simulink model "hw3"  (R2020a)
settings: Solver=VariableStepAuto  StartTime=0.0  StopTime=1  RelTol=1e-3
undefined symbols (not defined in the file): Beq, D2R, Gr, Jeq, Ka_c, Ka_s, Kd_p, Ke, Ki_c, Ki_s, Kp_c, Kp_p, Kp_s, Kt, La, Ra
(part 1 of 2)
settings Model: Creator=helep  LastModifiedBy=JeongHun Hong
settings SFSimCC: CustomCodeUndefinedFunction=UseInterfaceOnly

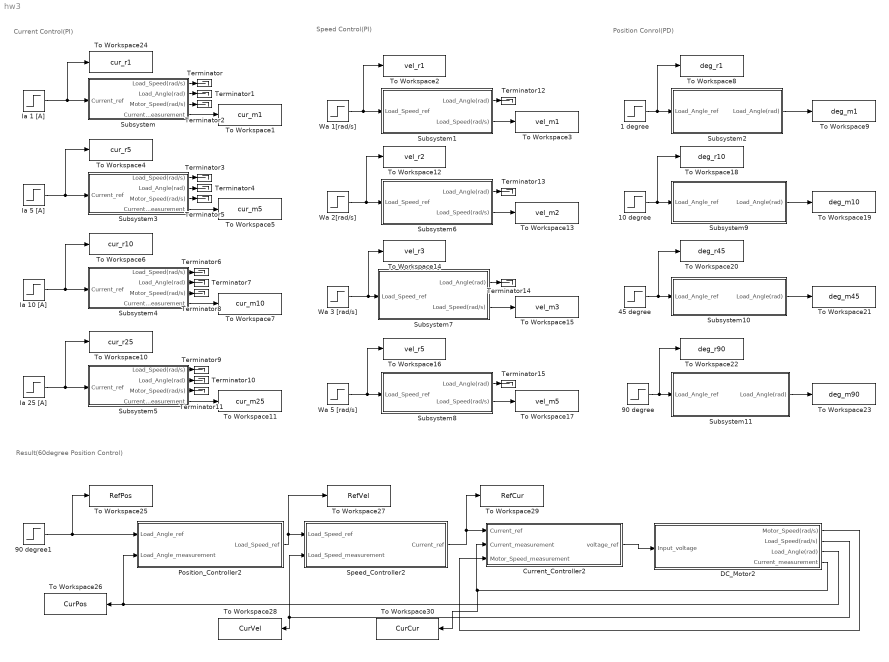
== system hw3 ==
  note: Position Conrol(PD)
  note: Speed Control(PI)
  note: Current Control(PI)
  note: Result(60degree Position Control)
  1 degree : Step  Time=0  After=1*D2R  SampleTime=0
  10 degree : Step  Time=0  After=10*D2R  SampleTime=0
  45 degree : Step  Time=0  After=45*D2R  SampleTime=0
  90 degree : Step  Time=0  After=90*D2R  SampleTime=0
  90 degree1 : Step  Time=0  After=60*D2R  SampleTime=0
  Current_Controller2 : Subsystem
  DC_Motor2 : Subsystem
  Ia 1 [A] : Step  Time=0  SampleTime=0
  Ia 10 [A] : Step  Time=0  After=10  SampleTime=0
  Ia 25 [A] : Step  Time=0  After=25  SampleTime=0
  Ia 5 [A] : Step  Time=0  After=5  SampleTime=0
  Position_Controller2 : Subsystem
  Speed_Controller2 : Subsystem
  Subsystem : Subsystem
  Subsystem1 : Subsystem
  Subsystem10 : Subsystem
  Subsystem11 : Subsystem
  Subsystem2 : Subsystem
  Subsystem3 : Subsystem
  Subsystem4 : Subsystem
  Subsystem5 : Subsystem
  Subsystem6 : Subsystem
  Subsystem7 : Subsystem
  Subsystem8 : Subsystem
  Subsystem9 : Subsystem
  Terminator{,1..15} (16 alike) : Terminator
  To Workspace1 : ToWorkspace  VariableName=cur_m1  SaveFormat=Structure With Time  SampleTime=-1
  To Workspace10 : ToWorkspace  VariableName=cur_r25  SaveFormat=Structure With Time  SampleTime=-1
  To Workspace11 : ToWorkspace  VariableName=cur_m25  SaveFormat=Structure With Time  SampleTime=-1
  To Workspace12 : ToWorkspace  VariableName=vel_r2  SaveFormat=Structure With Time  SampleTime=-1
  To Workspace13 : ToWorkspace  VariableName=vel_m2  SaveFormat=Structure With Time  SampleTime=-1
  To Workspace14 : ToWorkspace  VariableName=vel_r3  SaveFormat=Structure With Time  SampleTime=-1
  To Workspace15 : ToWorkspace  VariableName=vel_m3  SaveFormat=Structure With Time  SampleTime=-1
  To Workspace16 : ToWorkspace  VariableName=vel_r5  SaveFormat=Structure With Time  SampleTime=-1
  To Workspace17 : ToWorkspace  VariableName=vel_m5  SaveFormat=Structure With Time  SampleTime=-1
  To Workspace18 : ToWorkspace  VariableName=deg_r10  SaveFormat=Structure With Time  SampleTime=-1
  To Workspace19 : ToWorkspace  VariableName=deg_m10  SaveFormat=Structure With Time  SampleTime=-1
  To Workspace2 : ToWorkspace  VariableName=vel_r1  SaveFormat=Structure With Time  SampleTime=-1
  To Workspace20 : ToWorkspace  VariableName=deg_r45  SaveFormat=Structure With Time  SampleTime=-1
  To Workspace21 : ToWorkspace  VariableName=deg_m45  SaveFormat=Structure With Time  SampleTime=-1
  To Workspace22 : ToWorkspace  VariableName=deg_r90  SaveFormat=Structure With Time  SampleTime=-1
  To Workspace23 : ToWorkspace  VariableName=deg_m90  SaveFormat=Structure With Time  SampleTime=-1
  To Workspace24 : ToWorkspace  VariableName=cur_r1  SaveFormat=Structure With Time  SampleTime=-1
  To Workspace25 : ToWorkspace  VariableName=RefPos  SaveFormat=Structure With Time  SampleTime=-1
  To Workspace26 : ToWorkspace  VariableName=CurPos  SaveFormat=Structure With Time  SampleTime=-1
  To Workspace27 : ToWorkspace  VariableName=RefVel  SaveFormat=Structure With Time  SampleTime=-1
  To Workspace28 : ToWorkspace  VariableName=CurVel  SaveFormat=Structure With Time  SampleTime=-1
  To Workspace29 : ToWorkspace  VariableName=RefCur  SaveFormat=Structure With Time  SampleTime=-1
  To Workspace3 : ToWorkspace  VariableName=vel_m1  SaveFormat=Structure With Time  SampleTime=-1
  To Workspace30 : ToWorkspace  VariableName=CurCur  SaveFormat=Structure With Time  SampleTime=-1
  To Workspace4 : ToWorkspace  VariableName=cur_r5  SaveFormat=Structure With Time  SampleTime=-1
  To Workspace5 : ToWorkspace  VariableName=cur_m5  SaveFormat=Structure With Time  SampleTime=-1
  To Workspace6 : ToWorkspace  VariableName=cur_r10  SaveFormat=Structure With Time  SampleTime=-1
  To Workspace7 : ToWorkspace  VariableName=cur_m10  SaveFormat=Structure With Time  SampleTime=-1
  To Workspace8 : ToWorkspace  VariableName=deg_r1  SaveFormat=Structure With Time  SampleTime=-1
  To Workspace9 : ToWorkspace  VariableName=deg_m1  SaveFormat=Structure With Time  SampleTime=-1
  Wa 1[rad/s] : Step  Time=0  SampleTime=0
  Wa 2[rad/s] : Step  Time=0  After=2  SampleTime=0
  Wa 3 [rad/s] : Step  Time=0  After=3  SampleTime=0
  Wa 5 [rad/s] : Step  Time=0  After=5  SampleTime=0
  wires:
  Ia 1 [A]/1 -> To Workspace24/1, Subsystem/1(Current_ref)
  Wa 1[rad/s]/1 -> To Workspace2/1, Subsystem1/1(Load_Speed_ref)
  1 degree/1 -> To Workspace8/1, Subsystem2/1(Load_Angle_ref)
  Subsystem1/2(Load_Speed(rad/s)) -> To Workspace3/1
  Subsystem2/1(Load_Angle(rad)) -> To Workspace9/1
  Ia 5 [A]/1 -> To Workspace4/1, Subsystem3/1(Current_ref)
  Ia 10 [A]/1 -> To Workspace6/1, Subsystem4/1(Current_ref)
  Ia 25 [A]/1 -> To Workspace10/1, Subsystem5/1(Current_ref)
  Subsystem6/2(Load_Speed(rad/s)) -> To Workspace13/1
  Wa 2[rad/s]/1 -> To Workspace12/1, Subsystem6/1(Load_Speed_ref)
  Wa 3 [rad/s]/1 -> To Workspace14/1, Subsystem7/1(Load_Speed_ref)
  Wa 5 [rad/s]/1 -> To Workspace16/1, Subsystem8/1(Load_Speed_ref)
  Subsystem7/2(Load_Speed(rad/s)) -> To Workspace15/1
  Subsystem8/2(Load_Speed(rad/s)) -> To Workspace17/1
  10 degree/1 -> To Workspace18/1, Subsystem9/1(Load_Angle_ref)
  45 degree/1 -> To Workspace20/1, Subsystem10/1(Load_Angle_ref)
  90 degree/1 -> To Workspace22/1, Subsystem11/1(Load_Angle_ref)
  Subsystem9/1(Load_Angle(rad)) -> To Workspace19/1
  Subsystem10/1(Load_Angle(rad)) -> To Workspace21/1
  Subsystem11/1(Load_Angle(rad)) -> To Workspace23/1
  Subsystem/4(Current_measurement) -> To Workspace1/1
  Subsystem3/4(Current_measurement) -> To Workspace5/1
  Subsystem4/4(Current_measurement) -> To Workspace7/1
  Subsystem5/4(Current_measurement) -> To Workspace11/1
  Subsystem/1(Load_Speed(rad/s)) -> Terminator/1
  Subsystem/2(Load_Angle(rad)) -> Terminator1/1
  Subsystem/3(Motor_Speed(rad/s)) -> Terminator2/1
  Subsystem1/1(Load_Angle(rad)) -> Terminator12/1
  Subsystem6/1(Load_Angle(rad)) -> Terminator13/1
  Subsystem7/1(Load_Angle(rad)) -> Terminator14/1
  Subsystem8/1(Load_Angle(rad)) -> Terminator15/1
  Subsystem3/1(Load_Speed(rad/s)) -> Terminator3/1
  Subsystem3/2(Load_Angle(rad)) -> Terminator4/1
  Subsystem3/3(Motor_Speed(rad/s)) -> Terminator5/1
  Subsystem4/3(Motor_Speed(rad/s)) -> Terminator8/1
  Subsystem4/2(Load_Angle(rad)) -> Terminator7/1
  Subsystem4/1(Load_Speed(rad/s)) -> Terminator6/1
  Subsystem5/3(Motor_Speed(rad/s)) -> Terminator11/1
  Subsystem5/2(Load_Angle(rad)) -> Terminator10/1
  Subsystem5/1(Load_Speed(rad/s)) -> Terminator9/1
  DC_Motor2/3(Load_Angle(rad)) -> Position_Controller2/2(Load_Angle_measurement), To Workspace26/1
  Current_Controller2/1(voltage_ref) -> DC_Motor2/1(Input_voltage)
  Speed_Controller2/1(Current_ref) -> To Workspace29/1, Current_Controller2/1(Current_ref)
  DC_Motor2/2(Load_Speed(rad/s)) -> To Workspace28/1, Speed_Controller2/2(Load_Speed_measurement)
  DC_Motor2/1(Motor_Speed(rad/s)) -> Current_Controller2/3(Motor_Speed_measurement)
  DC_Motor2/4(Current_measurement) -> To Workspace30/1, Current_Controller2/2(Current_measurement)
  90 degree1/1 -> To Workspace25/1, Position_Controller2/1(Load_Angle_ref)
  Position_Controller2/1(Load_Speed_ref) -> To Workspace27/1, Speed_Controller2/1(Load_Speed_ref)

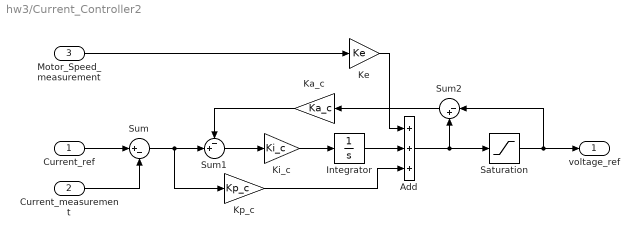
== system hw3/Current_Controller2 ==
  Current_ref : Inport
  Current_measurement : Inport  Port=2
  Motor_Speed_measurement : Inport  Port=3
  Add : Sum  Inputs=+++
  Integrator : Integrator
  Ka_c : Gain  Gain=Ka_c
  Ke : Gain  Gain=Ke
  Ki_c : Gain  Gain=Ki_c
  Kp_c : Gain  Gain=Kp_c
  Saturation : Saturate  UpperLimit=48  LowerLimit=-48
  Sum : Sum  Inputs=|+-
  Sum1 : Sum  Inputs=-+|
  Sum2 : Sum  Inputs=|-+
  voltage_ref : Outport  VectorParamsAs1DForOutWhenUnconnected=off
  wires:
  Saturation/1 -> Sum2/1, voltage_ref/1
  Ke/1 -> Add/1
  Motor_Speed_measurement/1 -> Ke/1
  Ka_c/1 -> Sum1/1
  Current_ref/1 -> Sum/1
  Current_measurement/1 -> Sum/2
  Sum1/1 -> Ki_c/1
  Integrator/1 -> Add/2
  Sum/1 -> Sum1/2, Kp_c/1
  Kp_c/1 -> Add/3
  Sum2/1 -> Ka_c/1
  Ki_c/1 -> Integrator/1
  Add/1 -> Sum2/2, Saturation/1

== system hw3/DC_Motor2 ==
  Input_voltage : Inport
  Back EMF constant1 : Gain  Gain=Ke
  Gr : Gain  Gain=Gr
  Integrator1 : Integrator
  Sum1 : Sum  Inputs=|+-
  Torque constant1 : Gain  Gain=Kt
  Transfer Fcn1 : TransferFcn  Denominator=[La Ra]
  Transfer Fcn3 : TransferFcn  Denominator=[Jeq Beq]
  Motor_Speed(rad/s) : Outport  VectorParamsAs1DForOutWhenUnconnected=off
  Load_Speed(rad/s) : Outport  Port=2  VectorParamsAs1DForOutWhenUnconnected=off
  Load_Angle(rad) : Outport  Port=3  VectorParamsAs1DForOutWhenUnconnected=off
  Current_measurement : Outport  Port=4  VectorParamsAs1DForOutWhenUnconnected=off
  wires:
  Transfer Fcn3/1 -> Back EMF constant1/1, Gr/1, Motor_Speed(rad/s)/1
  Integrator1/1 -> Load_Angle(rad)/1
  Gr/1 -> Integrator1/1, Load_Speed(rad/s)/1
  Input_voltage/1 -> Sum1/1
  Sum1/1 -> Transfer Fcn1/1
  Transfer Fcn1/1 -> Current_measurement/1, Torque constant1/1
  Back EMF constant1/1 -> Sum1/2
  Torque constant1/1 -> Transfer Fcn3/1

== system hw3/Position_Controller2 ==
  Load_Angle_ref : Inport
  Load_Angle_measurement : Inport  Port=2
  Add : Sum
  Derivative : Derivative
  Kd_p : Gain  Gain=Kd_p
  Kp_p : Gain  Gain=Kp_p
  Saturation : Saturate  UpperLimit=6140*pi/30  LowerLimit=-6140*pi/30
  Sum : Sum  Inputs=|+-
  Load_Speed_ref : Outport  VectorParamsAs1DForOutWhenUnconnected=off
  wires:
  Add/1 -> Saturation/1
  Derivative/1 -> Add/2
  Sum/1 -> Kd_p/1, Kp_p/1
  Saturation/1 -> Load_Speed_ref/1
  Kp_p/1 -> Add/1
  Kd_p/1 -> Derivative/1
  Load_Angle_ref/1 -> Sum/1
  Load_Angle_measurement/1 -> Sum/2

== system hw3/Speed_Controller2 ==
  Load_Speed_ref : Inport
  Load_Speed_measurement : Inport  Port=2
  Add : Sum
  Integrator : Integrator
  Ka_s : Gain  Gain=Ka_s
  Ki_s : Gain  Gain=Ki_s
  Kp_s : Gain  Gain=Kp_s
  Saturation : Saturate  UpperLimit=27.3  LowerLimit=-27.3
  Sum : Sum  Inputs=|+-
  Sum1 : Sum  Inputs=-+|
  Sum2 : Sum  Inputs=|-+
  Current_ref : Outport  VectorParamsAs1DForOutWhenUnconnected=off
  wires:
  Integrator/1 -> Add/1
  Sum1/1 -> Ki_s/1
  Ki_s/1 -> Integrator/1
  Saturation/1 -> Sum2/1, Current_ref/1
  Load_Speed_measurement/1 -> Sum/2
  Ka_s/1 -> Sum1/1
  Sum2/1 -> Ka_s/1
  Add/1 -> Saturation/1, Sum2/2
  Load_Speed_ref/1 -> Sum/1
  Kp_s/1 -> Add/2
  Sum/1 -> Sum1/2, Kp_s/1

== system hw3/Subsystem ==
  Current_ref : Inport
  Current_Controller : Subsystem
  DC_Motor : Subsystem
  Load_Speed(rad/s) : Outport
  Load_Angle(rad) : Outport  Port=2
  Motor_Speed(rad/s) : Outport  Port=3
  Current_measurement : Outport  Port=4
  wires:
  DC_Motor/1(Motor_Speed(rad/s)) -> Motor_Speed(rad/s)/1, Current_Controller/3(Motor_Speed_measurement)
  Current_ref/1 -> Current_Controller/1(Current_ref)
  DC_Motor/2(Load_Speed(rad/s)) -> Load_Speed(rad/s)/1
  Current_Controller/1(voltage_ref) -> DC_Motor/1(Input_voltage)
  DC_Motor/3(Load_Angle(rad)) -> Load_Angle(rad)/1
  DC_Motor/4(Current_measurement) -> Current_measurement/1, Current_Controller/2(Current_measurement)

== system hw3/Subsystem1 ==
  Load_Speed_ref : Inport
  Current_Controller1 : Subsystem
  DC_Motor1 : Subsystem
  Speed_Controller1 : Subsystem
  Load_Angle(rad) : Outport
  Load_Speed(rad/s) : Outport  Port=2
  wires:
  Current_Controller1/1(voltage_ref) -> DC_Motor1/1(Input_voltage)
  DC_Motor1/2(Load_Speed(rad/s)) -> Load_Speed(rad/s)/1, Speed_Controller1/2(Load_Speed_measurement)
  Speed_Controller1/1(Current_ref) -> Current_Controller1/1(Current_ref)
  Load_Speed_ref/1 -> Speed_Controller1/1(Load_Speed_ref)
  DC_Motor1/3(Load_Angle(rad)) -> Load_Angle(rad)/1
  DC_Motor1/4(Current_measurement) -> Current_Controller1/2(Current_measurement)
  DC_Motor1/1(Motor_Speed(rad/s)) -> Current_Controller1/3(Motor_Speed_measurement)

== system hw3/Subsystem10 ==
  Load_Angle_ref : Inport
  Current_Controller2 : Subsystem
  DC_Motor2 : Subsystem
  Position_Controller2 : Subsystem
  Speed_Controller2 : Subsystem
  Load_Angle(rad) : Outport
  wires:
  DC_Motor2/3(Load_Angle(rad)) -> Load_Angle(rad)/1, Position_Controller2/2(Load_Angle_measurement)
  Load_Angle_ref/1 -> Position_Controller2/1(Load_Angle_ref)
  Current_Controller2/1(voltage_ref) -> DC_Motor2/1(Input_voltage)
  Speed_Controller2/1(Current_ref) -> Current_Controller2/1(Current_ref)
  DC_Motor2/2(Load_Speed(rad/s)) -> Speed_Controller2/2(Load_Speed_measurement)
  Position_Controller2/1(Load_Speed_ref) -> Speed_Controller2/1(Load_Speed_ref)
  DC_Motor2/1(Motor_Speed(rad/s)) -> Current_Controller2/3(Motor_Speed_measurement)
  DC_Motor2/4(Current_measurement) -> Current_Controller2/2(Current_measurement)

== system hw3/Subsystem11 ==
  Load_Angle_ref : Inport
  Current_Controller2 : Subsystem
  DC_Motor2 : Subsystem
  Position_Controller2 : Subsystem
  Speed_Controller2 : Subsystem
  Load_Angle(rad) : Outport
  wires:
  DC_Motor2/4(Current_measurement) -> Current_Controller2/2(Current_measurement)
  DC_Motor2/1(Motor_Speed(rad/s)) -> Current_Controller2/3(Motor_Speed_measurement)
  Position_Controller2/1(Load_Speed_ref) -> Speed_Controller2/1(Load_Speed_ref)
  DC_Motor2/2(Load_Speed(rad/s)) -> Speed_Controller2/2(Load_Speed_measurement)
  Speed_Controller2/1(Current_ref) -> Current_Controller2/1(Current_ref)
  Current_Controller2/1(voltage_ref) -> DC_Motor2/1(Input_voltage)
  Load_Angle_ref/1 -> Position_Controller2/1(Load_Angle_ref)
  DC_Motor2/3(Load_Angle(rad)) -> Position_Controller2/2(Load_Angle_measurement), Load_Angle(rad)/1

== system hw3/Subsystem2 ==
  Load_Angle_ref : Inport
  Current_Controller2 : Subsystem
  DC_Motor2 : Subsystem
  Position_Controller2 : Subsystem
  Speed_Controller2 : Subsystem
  Load_Angle(rad) : Outport
  wires:
  DC_Motor2/3(Load_Angle(rad)) -> Load_Angle(rad)/1, Position_Controller2/2(Load_Angle_measurement)
  Load_Angle_ref/1 -> Position_Controller2/1(Load_Angle_ref)
  Current_Controller2/1(voltage_ref) -> DC_Motor2/1(Input_voltage)
  Speed_Controller2/1(Current_ref) -> Current_Controller2/1(Current_ref)
  DC_Motor2/2(Load_Speed(rad/s)) -> Speed_Controller2/2(Load_Speed_measurement)
  Position_Controller2/1(Load_Speed_ref) -> Speed_Controller2/1(Load_Speed_ref)
  DC_Motor2/1(Motor_Speed(rad/s)) -> Current_Controller2/3(Motor_Speed_measurement)
  DC_Motor2/4(Current_measurement) -> Current_Controller2/2(Current_measurement)

== system hw3/Subsystem3 ==
  Current_ref : Inport
  Current_Controller : Subsystem
  DC_Motor : Subsystem
  Load_Speed(rad/s) : Outport
  Load_Angle(rad) : Outport  Port=2
  Motor_Speed(rad/s) : Outport  Port=3
  Current_measurement : Outport  Port=4
  wires:
  DC_Motor/4(Current_measurement) -> Current_measurement/1, Current_Controller/2(Current_measurement)
  DC_Motor/3(Load_Angle(rad)) -> Load_Angle(rad)/1
  Current_Controller/1(voltage_ref) -> DC_Motor/1(Input_voltage)
  DC_Motor/2(Load_Speed(rad/s)) -> Load_Speed(rad/s)/1
  Current_ref/1 -> Current_Controller/1(Current_ref)
  DC_Motor/1(Motor_Speed(rad/s)) -> Current_Controller/3(Motor_Speed_measurement), Motor_Speed(rad/s)/1

== system hw3/Subsystem4 ==
  Current_ref : Inport
  Current_Controller : Subsystem
  DC_Motor : Subsystem
  Load_Speed(rad/s) : Outport
  Load_Angle(rad) : Outport  Port=2
  Motor_Speed(rad/s) : Outport  Port=3
  Current_measurement : Outport  Port=4
  wires:
  DC_Motor/1(Motor_Speed(rad/s)) -> Motor_Speed(rad/s)/1, Current_Controller/3(Motor_Speed_measurement)
  Current_ref/1 -> Current_Controller/1(Current_ref)
  DC_Motor/2(Load_Speed(rad/s)) -> Load_Speed(rad/s)/1
  Current_Controller/1(voltage_ref) -> DC_Motor/1(Input_voltage)
  DC_Motor/3(Load_Angle(rad)) -> Load_Angle(rad)/1
  DC_Motor/4(Current_measurement) -> Current_measurement/1, Current_Controller/2(Current_measurement)

== system hw3/Subsystem5 ==
  Current_ref : Inport
  Current_Controller : Subsystem
  DC_Motor : Subsystem
  Load_Speed(rad/s) : Outport
  Load_Angle(rad) : Outport  Port=2
  Motor_Speed(rad/s) : Outport  Port=3
  Current_measurement : Outport  Port=4
  wires:
  DC_Motor/4(Current_measurement) -> Current_measurement/1, Current_Controller/2(Current_measurement)
  DC_Motor/3(Load_Angle(rad)) -> Load_Angle(rad)/1
  Current_Controller/1(voltage_ref) -> DC_Motor/1(Input_voltage)
  DC_Motor/2(Load_Speed(rad/s)) -> Load_Speed(rad/s)/1
  Current_ref/1 -> Current_Controller/1(Current_ref)
  DC_Motor/1(Motor_Speed(rad/s)) -> Current_Controller/3(Motor_Speed_measurement), Motor_Speed(rad/s)/1

== system hw3/Subsystem6 ==
  Load_Speed_ref : Inport
  Current_Controller1 : Subsystem
  DC_Motor1 : Subsystem
  Speed_Controller1 : Subsystem
  Load_Angle(rad) : Outport
  Load_Speed(rad/s) : Outport  Port=2
  wires:
  DC_Motor1/1(Motor_Speed(rad/s)) -> Current_Controller1/3(Motor_Speed_measurement)
  DC_Motor1/4(Current_measurement) -> Current_Controller1/2(Current_measurement)
  DC_Motor1/3(Load_Angle(rad)) -> Load_Angle(rad)/1
  Load_Speed_ref/1 -> Speed_Controller1/1(Load_Speed_ref)
  Speed_Controller1/1(Current_ref) -> Current_Controller1/1(Current_ref)
  DC_Motor1/2(Load_Speed(rad/s)) -> Speed_Controller1/2(Load_Speed_measurement), Load_Speed(rad/s)/1
  Current_Controller1/1(voltage_ref) -> DC_Motor1/1(Input_voltage)

== system hw3/Subsystem7 ==
  Load_Speed_ref : Inport
  Current_Controller1 : Subsystem
  DC_Motor1 : Subsystem
  Speed_Controller1 : Subsystem
  Load_Angle(rad) : Outport
  Load_Speed(rad/s) : Outport  Port=2
  wires:
  Current_Controller1/1(voltage_ref) -> DC_Motor1/1(Input_voltage)
  DC_Motor1/2(Load_Speed(rad/s)) -> Load_Speed(rad/s)/1, Speed_Controller1/2(Load_Speed_measurement)
  Speed_Controller1/1(Current_ref) -> Current_Controller1/1(Current_ref)
  Load_Speed_ref/1 -> Speed_Controller1/1(Load_Speed_ref)
  DC_Motor1/3(Load_Angle(rad)) -> Load_Angle(rad)/1
  DC_Motor1/4(Current_measurement) -> Current_Controller1/2(Current_measurement)
  DC_Motor1/1(Motor_Speed(rad/s)) -> Current_Controller1/3(Motor_Speed_measurement)

== system hw3/Subsystem8 ==
  Load_Speed_ref : Inport
  Current_Controller1 : Subsystem
  DC_Motor1 : Subsystem
  Speed_Controller1 : Subsystem
  Load_Angle(rad) : Outport
  Load_Speed(rad/s) : Outport  Port=2
  wires:
  DC_Motor1/1(Motor_Speed(rad/s)) -> Current_Controller1/3(Motor_Speed_measurement)
  DC_Motor1/4(Current_measurement) -> Current_Controller1/2(Current_measurement)
  DC_Motor1/3(Load_Angle(rad)) -> Load_Angle(rad)/1
  Load_Speed_ref/1 -> Speed_Controller1/1(Load_Speed_ref)
  Speed_Controller1/1(Current_ref) -> Current_Controller1/1(Current_ref)
  DC_Motor1/2(Load_Speed(rad/s)) -> Speed_Controller1/2(Load_Speed_measurement), Load_Speed(rad/s)/1
  Current_Controller1/1(voltage_ref) -> DC_Motor1/1(Input_voltage)

== system hw3/Subsystem9 ==
  Load_Angle_ref : Inport
  Current_Controller2 : Subsystem
  DC_Motor2 : Subsystem
  Position_Controller2 : Subsystem
  Speed_Controller2 : Subsystem
  Load_Angle(rad) : Outport
  wires:
  DC_Motor2/4(Current_measurement) -> Current_Controller2/2(Current_measurement)
  DC_Motor2/1(Motor_Speed(rad/s)) -> Current_Controller2/3(Motor_Speed_measurement)
  Position_Controller2/1(Load_Speed_ref) -> Speed_Controller2/1(Load_Speed_ref)
  DC_Motor2/2(Load_Speed(rad/s)) -> Speed_Controller2/2(Load_Speed_measurement)
  Speed_Controller2/1(Current_ref) -> Current_Controller2/1(Current_ref)
  Current_Controller2/1(voltage_ref) -> DC_Motor2/1(Input_voltage)
  Load_Angle_ref/1 -> Position_Controller2/1(Load_Angle_ref)
  DC_Motor2/3(Load_Angle(rad)) -> Position_Controller2/2(Load_Angle_measurement), Load_Angle(rad)/1

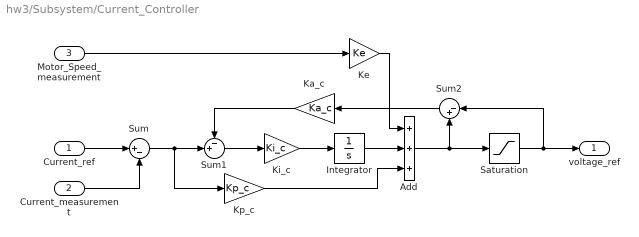
== system hw3/Subsystem/Current_Controller ==
  Current_ref : Inport
  Current_measurement : Inport  Port=2
  Motor_Speed_measurement : Inport  Port=3
  Add : Sum  Inputs=+++
  Integrator : Integrator
  Ka_c : Gain  Gain=Ka_c
  Ke : Gain  Gain=Ke
  Ki_c : Gain  Gain=Ki_c
  Kp_c : Gain  Gain=Kp_c
  Saturation : Saturate  UpperLimit=48  LowerLimit=-48
  Sum : Sum  Inputs=|+-
  Sum1 : Sum  Inputs=-+|
  Sum2 : Sum  Inputs=|-+
  voltage_ref : Outport  VectorParamsAs1DForOutWhenUnconnected=off
  wires:
  Add/1 -> Saturation/1, Sum2/2
  Ki_c/1 -> Integrator/1
  Sum2/1 -> Ka_c/1
  Kp_c/1 -> Add/3
  Sum/1 -> Kp_c/1, Sum1/2
  Integrator/1 -> Add/2
  Sum1/1 -> Ki_c/1
  Current_measurement/1 -> Sum/2
  Current_ref/1 -> Sum/1
  Ka_c/1 -> Sum1/1
  Motor_Speed_measurement/1 -> Ke/1
  Ke/1 -> Add/1
  Saturation/1 -> voltage_ref/1, Sum2/1

== system hw3/Subsystem/DC_Motor ==
  Input_voltage : Inport
  Back EMF constant1 : Gain  Gain=Ke
  Gr : Gain  Gain=Gr
  Integrator1 : Integrator
  Sum1 : Sum  Inputs=|+-
  Torque constant1 : Gain  Gain=Kt
  Transfer Fcn1 : TransferFcn  Denominator=[La Ra]
  Transfer Fcn3 : TransferFcn  Denominator=[Jeq Beq]
  Motor_Speed(rad/s) : Outport  VectorParamsAs1DForOutWhenUnconnected=off
  Load_Speed(rad/s) : Outport  Port=2  VectorParamsAs1DForOutWhenUnconnected=off
  Load_Angle(rad) : Outport  Port=3  VectorParamsAs1DForOutWhenUnconnected=off
  Current_measurement : Outport  Port=4  VectorParamsAs1DForOutWhenUnconnected=off
  wires:
  Torque constant1/1 -> Transfer Fcn3/1
  Back EMF constant1/1 -> Sum1/2
  Transfer Fcn1/1 -> Torque constant1/1, Current_measurement/1
  Sum1/1 -> Transfer Fcn1/1
  Input_voltage/1 -> Sum1/1
  Gr/1 -> Load_Speed(rad/s)/1, Integrator1/1
  Integrator1/1 -> Load_Angle(rad)/1
  Transfer Fcn3/1 -> Motor_Speed(rad/s)/1, Gr/1, Back EMF constant1/1

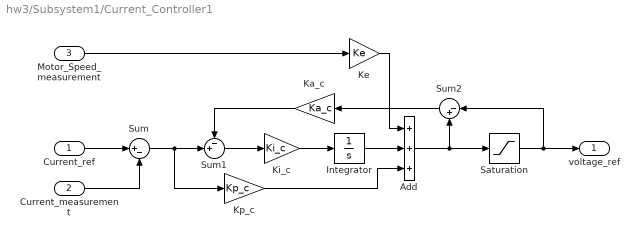
== system hw3/Subsystem1/Current_Controller1 ==
  Current_ref : Inport
  Current_measurement : Inport  Port=2
  Motor_Speed_measurement : Inport  Port=3
  Add : Sum  Inputs=+++
  Integrator : Integrator
  Ka_c : Gain  Gain=Ka_c
  Ke : Gain  Gain=Ke
  Ki_c : Gain  Gain=Ki_c
  Kp_c : Gain  Gain=Kp_c
  Saturation : Saturate  UpperLimit=48  LowerLimit=-48
  Sum : Sum  Inputs=|+-
  Sum1 : Sum  Inputs=-+|
  Sum2 : Sum  Inputs=|-+
  voltage_ref : Outport  VectorParamsAs1DForOutWhenUnconnected=off
  wires:
  Saturation/1 -> Sum2/1, voltage_ref/1
  Ke/1 -> Add/1
  Motor_Speed_measurement/1 -> Ke/1
  Ka_c/1 -> Sum1/1
  Current_ref/1 -> Sum/1
  Current_measurement/1 -> Sum/2
  Sum1/1 -> Ki_c/1
  Integrator/1 -> Add/2
  Sum/1 -> Sum1/2, Kp_c/1
  Kp_c/1 -> Add/3
  Sum2/1 -> Ka_c/1
  Ki_c/1 -> Integrator/1
  Add/1 -> Sum2/2, Saturation/1

== system hw3/Subsystem1/DC_Motor1 ==
  Input_voltage : Inport
  Back EMF constant1 : Gain  Gain=Ke
  Gr : Gain  Gain=Gr
  Integrator1 : Integrator
  Sum1 : Sum  Inputs=|+-
  Torque constant1 : Gain  Gain=Kt
  Transfer Fcn1 : TransferFcn  Denominator=[La Ra]
  Transfer Fcn3 : TransferFcn  Denominator=[Jeq Beq]
  Motor_Speed(rad/s) : Outport  VectorParamsAs1DForOutWhenUnconnected=off
  Load_Speed(rad/s) : Outport  Port=2  VectorParamsAs1DForOutWhenUnconnected=off
  Load_Angle(rad) : Outport  Port=3  VectorParamsAs1DForOutWhenUnconnected=off
  Current_measurement : Outport  Port=4  VectorParamsAs1DForOutWhenUnconnected=off
  wires:
  Transfer Fcn3/1 -> Back EMF constant1/1, Gr/1, Motor_Speed(rad/s)/1
  Integrator1/1 -> Load_Angle(rad)/1
  Gr/1 -> Integrator1/1, Load_Speed(rad/s)/1
  Input_voltage/1 -> Sum1/1
  Sum1/1 -> Transfer Fcn1/1
  Transfer Fcn1/1 -> Current_measurement/1, Torque constant1/1
  Back EMF constant1/1 -> Sum1/2
  Torque constant1/1 -> Transfer Fcn3/1

== system hw3/Subsystem1/Speed_Controller1 ==
  Load_Speed_ref : Inport
  Load_Speed_measurement : Inport  Port=2
  Add : Sum
  Integrator : Integrator
  Ka_s : Gain  Gain=Ka_s
  Ki_s : Gain  Gain=Ki_s
  Kp_s : Gain  Gain=Kp_s
  Saturation : Saturate  UpperLimit=27.3  LowerLimit=-27.3
  Sum : Sum  Inputs=|+-
  Sum1 : Sum  Inputs=-+|
  Sum2 : Sum  Inputs=|-+
  Current_ref : Outport  VectorParamsAs1DForOutWhenUnconnected=off
  wires:
  Integrator/1 -> Add/1
  Sum1/1 -> Ki_s/1
  Ki_s/1 -> Integrator/1
  Saturation/1 -> Sum2/1, Current_ref/1
  Load_Speed_measurement/1 -> Sum/2
  Ka_s/1 -> Sum1/1
  Sum2/1 -> Ka_s/1
  Add/1 -> Saturation/1, Sum2/2
  Load_Speed_ref/1 -> Sum/1
  Kp_s/1 -> Add/2
  Sum/1 -> Sum1/2, Kp_s/1

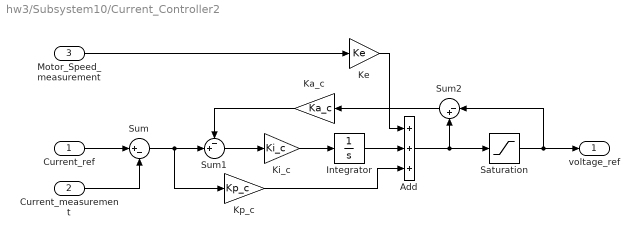
== system hw3/Subsystem10/Current_Controller2 ==
  Current_ref : Inport
  Current_measurement : Inport  Port=2
  Motor_Speed_measurement : Inport  Port=3
  Add : Sum  Inputs=+++
  Integrator : Integrator
  Ka_c : Gain  Gain=Ka_c
  Ke : Gain  Gain=Ke
  Ki_c : Gain  Gain=Ki_c
  Kp_c : Gain  Gain=Kp_c
  Saturation : Saturate  UpperLimit=48  LowerLimit=-48
  Sum : Sum  Inputs=|+-
  Sum1 : Sum  Inputs=-+|
  Sum2 : Sum  Inputs=|-+
  voltage_ref : Outport  VectorParamsAs1DForOutWhenUnconnected=off
  wires:
  Add/1 -> Saturation/1, Sum2/2
  Ki_c/1 -> Integrator/1
  Sum2/1 -> Ka_c/1
  Kp_c/1 -> Add/3
  Sum/1 -> Kp_c/1, Sum1/2
  Integrator/1 -> Add/2
  Sum1/1 -> Ki_c/1
  Current_measurement/1 -> Sum/2
  Current_ref/1 -> Sum/1
  Ka_c/1 -> Sum1/1
  Motor_Speed_measurement/1 -> Ke/1
  Ke/1 -> Add/1
  Saturation/1 -> voltage_ref/1, Sum2/1

== system hw3/Subsystem10/DC_Motor2 ==
  Input_voltage : Inport
  Back EMF constant1 : Gain  Gain=Ke
  Gr : Gain  Gain=Gr
  Integrator1 : Integrator
  Sum1 : Sum  Inputs=|+-
  Torque constant1 : Gain  Gain=Kt
  Transfer Fcn1 : TransferFcn  Denominator=[La Ra]
  Transfer Fcn3 : TransferFcn  Denominator=[Jeq Beq]
  Motor_Speed(rad/s) : Outport  VectorParamsAs1DForOutWhenUnconnected=off
  Load_Speed(rad/s) : Outport  Port=2  VectorParamsAs1DForOutWhenUnconnected=off
  Load_Angle(rad) : Outport  Port=3  VectorParamsAs1DForOutWhenUnconnected=off
  Current_measurement : Outport  Port=4  VectorParamsAs1DForOutWhenUnconnected=off
  wires:
  Torque constant1/1 -> Transfer Fcn3/1
  Back EMF constant1/1 -> Sum1/2
  Transfer Fcn1/1 -> Torque constant1/1, Current_measurement/1
  Sum1/1 -> Transfer Fcn1/1
  Input_voltage/1 -> Sum1/1
  Gr/1 -> Load_Speed(rad/s)/1, Integrator1/1
  Integrator1/1 -> Load_Angle(rad)/1
  Transfer Fcn3/1 -> Motor_Speed(rad/s)/1, Gr/1, Back EMF constant1/1

== system hw3/Subsystem10/Position_Controller2 ==
  Load_Angle_ref : Inport
  Load_Angle_measurement : Inport  Port=2
  Add : Sum
  Derivative : Derivative
  Kd_p : Gain  Gain=Kd_p
  Kp_p : Gain  Gain=Kp_p
  Saturation : Saturate  UpperLimit=6140*pi/30  LowerLimit=-6140*pi/30
  Sum : Sum  Inputs=|+-
  Load_Speed_ref : Outport  VectorParamsAs1DForOutWhenUnconnected=off
  wires:
  Load_Angle_measurement/1 -> Sum/2
  Load_Angle_ref/1 -> Sum/1
  Kd_p/1 -> Derivative/1
  Kp_p/1 -> Add/1
  Saturation/1 -> Load_Speed_ref/1
  Sum/1 -> Kp_p/1, Kd_p/1
  Derivative/1 -> Add/2
  Add/1 -> Saturation/1

== system hw3/Subsystem10/Speed_Controller2 ==
  Load_Speed_ref : Inport
  Load_Speed_measurement : Inport  Port=2
  Add : Sum
  Integrator : Integrator
  Ka_s : Gain  Gain=Ka_s
  Ki_s : Gain  Gain=Ki_s
  Kp_s : Gain  Gain=Kp_s
  Saturation : Saturate  UpperLimit=27.3  LowerLimit=-27.3
  Sum : Sum  Inputs=|+-
  Sum1 : Sum  Inputs=-+|
  Sum2 : Sum  Inputs=|-+
  Current_ref : Outport  VectorParamsAs1DForOutWhenUnconnected=off
  wires:
  Sum/1 -> Kp_s/1, Sum1/2
  Kp_s/1 -> Add/2
  Load_Speed_ref/1 -> Sum/1
  Add/1 -> Sum2/2, Saturation/1
  Sum2/1 -> Ka_s/1
  Ka_s/1 -> Sum1/1
  Load_Speed_measurement/1 -> Sum/2
  Saturation/1 -> Current_ref/1, Sum2/1
  Ki_s/1 -> Integrator/1
  Sum1/1 -> Ki_s/1
  Integrator/1 -> Add/1

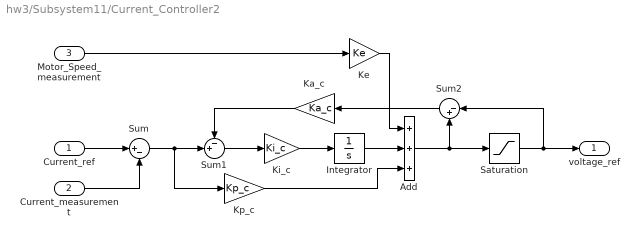
== system hw3/Subsystem11/Current_Controller2 ==
  Current_ref : Inport
  Current_measurement : Inport  Port=2
  Motor_Speed_measurement : Inport  Port=3
  Add : Sum  Inputs=+++
  Integrator : Integrator
  Ka_c : Gain  Gain=Ka_c
  Ke : Gain  Gain=Ke
  Ki_c : Gain  Gain=Ki_c
  Kp_c : Gain  Gain=Kp_c
  Saturation : Saturate  UpperLimit=48  LowerLimit=-48
  Sum : Sum  Inputs=|+-
  Sum1 : Sum  Inputs=-+|
  Sum2 : Sum  Inputs=|-+
  voltage_ref : Outport  VectorParamsAs1DForOutWhenUnconnected=off
  wires:
  Saturation/1 -> Sum2/1, voltage_ref/1
  Ke/1 -> Add/1
  Motor_Speed_measurement/1 -> Ke/1
  Ka_c/1 -> Sum1/1
  Current_ref/1 -> Sum/1
  Current_measurement/1 -> Sum/2
  Sum1/1 -> Ki_c/1
  Integrator/1 -> Add/2
  Sum/1 -> Sum1/2, Kp_c/1
  Kp_c/1 -> Add/3
  Sum2/1 -> Ka_c/1
  Ki_c/1 -> Integrator/1
  Add/1 -> Sum2/2, Saturation/1

== system hw3/Subsystem11/DC_Motor2 ==
  Input_voltage : Inport
  Back EMF constant1 : Gain  Gain=Ke
  Gr : Gain  Gain=Gr
  Integrator1 : Integrator
  Sum1 : Sum  Inputs=|+-
  Torque constant1 : Gain  Gain=Kt
  Transfer Fcn1 : TransferFcn  Denominator=[La Ra]
  Transfer Fcn3 : TransferFcn  Denominator=[Jeq Beq]
  Motor_Speed(rad/s) : Outport  VectorParamsAs1DForOutWhenUnconnected=off
  Load_Speed(rad/s) : Outport  Port=2  VectorParamsAs1DForOutWhenUnconnected=off
  Load_Angle(rad) : Outport  Port=3  VectorParamsAs1DForOutWhenUnconnected=off
  Current_measurement : Outport  Port=4  VectorParamsAs1DForOutWhenUnconnected=off
  wires:
  Transfer Fcn3/1 -> Back EMF constant1/1, Gr/1, Motor_Speed(rad/s)/1
  Integrator1/1 -> Load_Angle(rad)/1
  Gr/1 -> Integrator1/1, Load_Speed(rad/s)/1
  Input_voltage/1 -> Sum1/1
  Sum1/1 -> Transfer Fcn1/1
  Transfer Fcn1/1 -> Current_measurement/1, Torque constant1/1
  Back EMF constant1/1 -> Sum1/2
  Torque constant1/1 -> Transfer Fcn3/1

== system hw3/Subsystem11/Position_Controller2 ==
  Load_Angle_ref : Inport
  Load_Angle_measurement : Inport  Port=2
  Add : Sum
  Derivative : Derivative
  Kd_p : Gain  Gain=Kd_p
  Kp_p : Gain  Gain=Kp_p
  Saturation : Saturate  UpperLimit=6140*pi/30  LowerLimit=-6140*pi/30
  Sum : Sum  Inputs=|+-
  Load_Speed_ref : Outport  VectorParamsAs1DForOutWhenUnconnected=off
  wires:
  Add/1 -> Saturation/1
  Derivative/1 -> Add/2
  Sum/1 -> Kd_p/1, Kp_p/1
  Saturation/1 -> Load_Speed_ref/1
  Kp_p/1 -> Add/1
  Kd_p/1 -> Derivative/1
  Load_Angle_ref/1 -> Sum/1
  Load_Angle_measurement/1 -> Sum/2

== system hw3/Subsystem11/Speed_Controller2 ==
  Load_Speed_ref : Inport
  Load_Speed_measurement : Inport  Port=2
  Add : Sum
  Integrator : Integrator
  Ka_s : Gain  Gain=Ka_s
  Ki_s : Gain  Gain=Ki_s
  Kp_s : Gain  Gain=Kp_s
  Saturation : Saturate  UpperLimit=27.3  LowerLimit=-27.3
  Sum : Sum  Inputs=|+-
  Sum1 : Sum  Inputs=-+|
  Sum2 : Sum  Inputs=|-+
  Current_ref : Outport  VectorParamsAs1DForOutWhenUnconnected=off
  wires:
  Integrator/1 -> Add/1
  Sum1/1 -> Ki_s/1
  Ki_s/1 -> Integrator/1
  Saturation/1 -> Sum2/1, Current_ref/1
  Load_Speed_measurement/1 -> Sum/2
  Ka_s/1 -> Sum1/1
  Sum2/1 -> Ka_s/1
  Add/1 -> Saturation/1, Sum2/2
  Load_Speed_ref/1 -> Sum/1
  Kp_s/1 -> Add/2
  Sum/1 -> Sum1/2, Kp_s/1

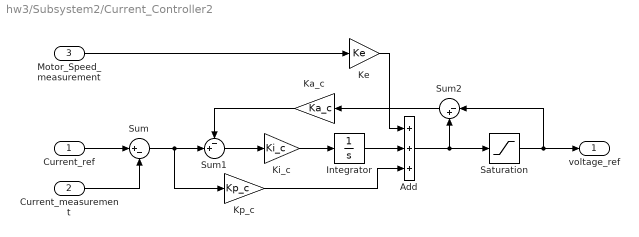
== system hw3/Subsystem2/Current_Controller2 ==
  Current_ref : Inport
  Current_measurement : Inport  Port=2
  Motor_Speed_measurement : Inport  Port=3
  Add : Sum  Inputs=+++
  Integrator : Integrator
  Ka_c : Gain  Gain=Ka_c
  Ke : Gain  Gain=Ke
  Ki_c : Gain  Gain=Ki_c
  Kp_c : Gain  Gain=Kp_c
  Saturation : Saturate  UpperLimit=48  LowerLimit=-48
  Sum : Sum  Inputs=|+-
  Sum1 : Sum  Inputs=-+|
  Sum2 : Sum  Inputs=|-+
  voltage_ref : Outport  VectorParamsAs1DForOutWhenUnconnected=off
  wires:
  Add/1 -> Saturation/1, Sum2/2
  Ki_c/1 -> Integrator/1
  Sum2/1 -> Ka_c/1
  Kp_c/1 -> Add/3
  Sum/1 -> Kp_c/1, Sum1/2
  Integrator/1 -> Add/2
  Sum1/1 -> Ki_c/1
  Current_measurement/1 -> Sum/2
  Current_ref/1 -> Sum/1
  Ka_c/1 -> Sum1/1
  Motor_Speed_measurement/1 -> Ke/1
  Ke/1 -> Add/1
  Saturation/1 -> voltage_ref/1, Sum2/1

== system hw3/Subsystem2/DC_Motor2 ==
  Input_voltage : Inport
  Back EMF constant1 : Gain  Gain=Ke
  Gr : Gain  Gain=Gr
  Integrator1 : Integrator
  Sum1 : Sum  Inputs=|+-
  Torque constant1 : Gain  Gain=Kt
  Transfer Fcn1 : TransferFcn  Denominator=[La Ra]
  Transfer Fcn3 : TransferFcn  Denominator=[Jeq Beq]
  Motor_Speed(rad/s) : Outport  VectorParamsAs1DForOutWhenUnconnected=off
  Load_Speed(rad/s) : Outport  Port=2  VectorParamsAs1DForOutWhenUnconnected=off
  Load_Angle(rad) : Outport  Port=3  VectorParamsAs1DForOutWhenUnconnected=off
  Current_measurement : Outport  Port=4  VectorParamsAs1DForOutWhenUnconnected=off
  wires:
  Torque constant1/1 -> Transfer Fcn3/1
  Back EMF constant1/1 -> Sum1/2
  Transfer Fcn1/1 -> Torque constant1/1, Current_measurement/1
  Sum1/1 -> Transfer Fcn1/1
  Input_voltage/1 -> Sum1/1
  Gr/1 -> Load_Speed(rad/s)/1, Integrator1/1
  Integrator1/1 -> Load_Angle(rad)/1
  Transfer Fcn3/1 -> Motor_Speed(rad/s)/1, Gr/1, Back EMF constant1/1

== system hw3/Subsystem2/Position_Controller2 ==
  Load_Angle_ref : Inport
  Load_Angle_measurement : Inport  Port=2
  Add : Sum
  Derivative : Derivative
  Kd_p : Gain  Gain=Kd_p
  Kp_p : Gain  Gain=Kp_p
  Saturation : Saturate  UpperLimit=6140*pi/30  LowerLimit=-6140*pi/30
  Sum : Sum  Inputs=|+-
  Load_Speed_ref : Outport  VectorParamsAs1DForOutWhenUnconnected=off
  wires:
  Load_Angle_measurement/1 -> Sum/2
  Load_Angle_ref/1 -> Sum/1
  Kd_p/1 -> Derivative/1
  Kp_p/1 -> Add/1
  Saturation/1 -> Load_Speed_ref/1
  Sum/1 -> Kp_p/1, Kd_p/1
  Derivative/1 -> Add/2
  Add/1 -> Saturation/1

== system hw3/Subsystem2/Speed_Controller2 ==
  Load_Speed_ref : Inport
  Load_Speed_measurement : Inport  Port=2
  Add : Sum
  Integrator : Integrator
  Ka_s : Gain  Gain=Ka_s
  Ki_s : Gain  Gain=Ki_s
  Kp_s : Gain  Gain=Kp_s
  Saturation : Saturate  UpperLimit=27.3  LowerLimit=-27.3
  Sum : Sum  Inputs=|+-
  Sum1 : Sum  Inputs=-+|
  Sum2 : Sum  Inputs=|-+
  Current_ref : Outport  VectorParamsAs1DForOutWhenUnconnected=off
  wires:
  Sum/1 -> Kp_s/1, Sum1/2
  Kp_s/1 -> Add/2
  Load_Speed_ref/1 -> Sum/1
  Add/1 -> Sum2/2, Saturation/1
  Sum2/1 -> Ka_s/1
  Ka_s/1 -> Sum1/1
  Load_Speed_measurement/1 -> Sum/2
  Saturation/1 -> Current_ref/1, Sum2/1
  Ki_s/1 -> Integrator/1
  Sum1/1 -> Ki_s/1
  Integrator/1 -> Add/1

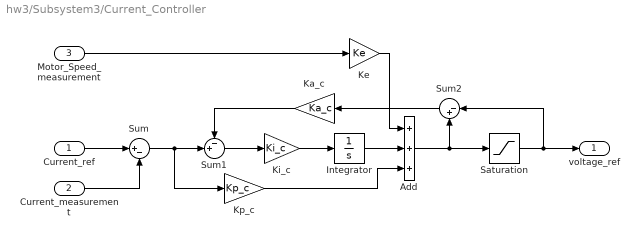
== system hw3/Subsystem3/Current_Controller ==
  Current_ref : Inport
  Current_measurement : Inport  Port=2
  Motor_Speed_measurement : Inport  Port=3
  Add : Sum  Inputs=+++
  Integrator : Integrator
  Ka_c : Gain  Gain=Ka_c
  Ke : Gain  Gain=Ke
  Ki_c : Gain  Gain=Ki_c
  Kp_c : Gain  Gain=Kp_c
  Saturation : Saturate  UpperLimit=48  LowerLimit=-48
  Sum : Sum  Inputs=|+-
  Sum1 : Sum  Inputs=-+|
  Sum2 : Sum  Inputs=|-+
  voltage_ref : Outport  VectorParamsAs1DForOutWhenUnconnected=off
  wires:
  Saturation/1 -> Sum2/1, voltage_ref/1
  Ke/1 -> Add/1
  Motor_Speed_measurement/1 -> Ke/1
  Ka_c/1 -> Sum1/1
  Current_ref/1 -> Sum/1
  Current_measurement/1 -> Sum/2
  Sum1/1 -> Ki_c/1
  Integrator/1 -> Add/2
  Sum/1 -> Sum1/2, Kp_c/1
  Kp_c/1 -> Add/3
  Sum2/1 -> Ka_c/1
  Ki_c/1 -> Integrator/1
  Add/1 -> Sum2/2, Saturation/1

== system hw3/Subsystem3/DC_Motor ==
  Input_voltage : Inport
  Back EMF constant1 : Gain  Gain=Ke
  Gr : Gain  Gain=Gr
  Integrator1 : Integrator
  Sum1 : Sum  Inputs=|+-
  Torque constant1 : Gain  Gain=Kt
  Transfer Fcn1 : TransferFcn  Denominator=[La Ra]
  Transfer Fcn3 : TransferFcn  Denominator=[Jeq Beq]
  Motor_Speed(rad/s) : Outport  VectorParamsAs1DForOutWhenUnconnected=off
  Load_Speed(rad/s) : Outport  Port=2  VectorParamsAs1DForOutWhenUnconnected=off
  Load_Angle(rad) : Outport  Port=3  VectorParamsAs1DForOutWhenUnconnected=off
  Current_measurement : Outport  Port=4  VectorParamsAs1DForOutWhenUnconnected=off
  wires:
  Transfer Fcn3/1 -> Back EMF constant1/1, Gr/1, Motor_Speed(rad/s)/1
  Integrator1/1 -> Load_Angle(rad)/1
  Gr/1 -> Integrator1/1, Load_Speed(rad/s)/1
  Input_voltage/1 -> Sum1/1
  Sum1/1 -> Transfer Fcn1/1
  Transfer Fcn1/1 -> Current_measurement/1, Torque constant1/1
  Back EMF constant1/1 -> Sum1/2
  Torque constant1/1 -> Transfer Fcn3/1

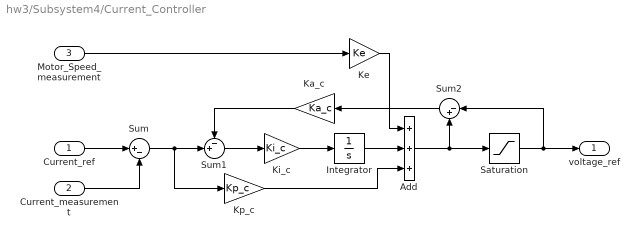
== system hw3/Subsystem4/Current_Controller ==
  Current_ref : Inport
  Current_measurement : Inport  Port=2
  Motor_Speed_measurement : Inport  Port=3
  Add : Sum  Inputs=+++
  Integrator : Integrator
  Ka_c : Gain  Gain=Ka_c
  Ke : Gain  Gain=Ke
  Ki_c : Gain  Gain=Ki_c
  Kp_c : Gain  Gain=Kp_c
  Saturation : Saturate  UpperLimit=48  LowerLimit=-48
  Sum : Sum  Inputs=|+-
  Sum1 : Sum  Inputs=-+|
  Sum2 : Sum  Inputs=|-+
  voltage_ref : Outport  VectorParamsAs1DForOutWhenUnconnected=off
  wires:
  Add/1 -> Saturation/1, Sum2/2
  Ki_c/1 -> Integrator/1
  Sum2/1 -> Ka_c/1
  Kp_c/1 -> Add/3
  Sum/1 -> Kp_c/1, Sum1/2
  Integrator/1 -> Add/2
  Sum1/1 -> Ki_c/1
  Current_measurement/1 -> Sum/2
  Current_ref/1 -> Sum/1
  Ka_c/1 -> Sum1/1
  Motor_Speed_measurement/1 -> Ke/1
  Ke/1 -> Add/1
  Saturation/1 -> voltage_ref/1, Sum2/1

== system hw3/Subsystem4/DC_Motor ==
  Input_voltage : Inport
  Back EMF constant1 : Gain  Gain=Ke
  Gr : Gain  Gain=Gr
  Integrator1 : Integrator
  Sum1 : Sum  Inputs=|+-
  Torque constant1 : Gain  Gain=Kt
  Transfer Fcn1 : TransferFcn  Denominator=[La Ra]
  Transfer Fcn3 : TransferFcn  Denominator=[Jeq Beq]
  Motor_Speed(rad/s) : Outport  VectorParamsAs1DForOutWhenUnconnected=off
  Load_Speed(rad/s) : Outport  Port=2  VectorParamsAs1DForOutWhenUnconnected=off
  Load_Angle(rad) : Outport  Port=3  VectorParamsAs1DForOutWhenUnconnected=off
  Current_measurement : Outport  Port=4  VectorParamsAs1DForOutWhenUnconnected=off
  wires:
  Torque constant1/1 -> Transfer Fcn3/1
  Back EMF constant1/1 -> Sum1/2
  Transfer Fcn1/1 -> Torque constant1/1, Current_measurement/1
  Sum1/1 -> Transfer Fcn1/1
  Input_voltage/1 -> Sum1/1
  Gr/1 -> Load_Speed(rad/s)/1, Integrator1/1
  Integrator1/1 -> Load_Angle(rad)/1
  Transfer Fcn3/1 -> Motor_Speed(rad/s)/1, Gr/1, Back EMF constant1/1

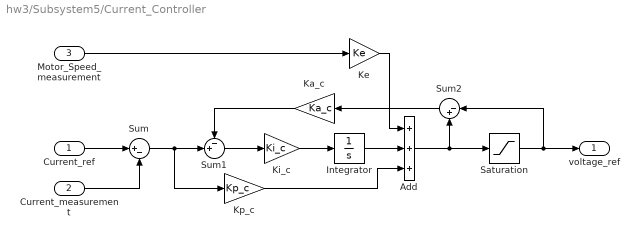
== system hw3/Subsystem5/Current_Controller ==
  Current_ref : Inport
  Current_measurement : Inport  Port=2
  Motor_Speed_measurement : Inport  Port=3
  Add : Sum  Inputs=+++
  Integrator : Integrator
  Ka_c : Gain  Gain=Ka_c
  Ke : Gain  Gain=Ke
  Ki_c : Gain  Gain=Ki_c
  Kp_c : Gain  Gain=Kp_c
  Saturation : Saturate  UpperLimit=48  LowerLimit=-48
  Sum : Sum  Inputs=|+-
  Sum1 : Sum  Inputs=-+|
  Sum2 : Sum  Inputs=|-+
  voltage_ref : Outport  VectorParamsAs1DForOutWhenUnconnected=off
  wires:
  Saturation/1 -> Sum2/1, voltage_ref/1
  Ke/1 -> Add/1
  Motor_Speed_measurement/1 -> Ke/1
  Ka_c/1 -> Sum1/1
  Current_ref/1 -> Sum/1
  Current_measurement/1 -> Sum/2
  Sum1/1 -> Ki_c/1
  Integrator/1 -> Add/2
  Sum/1 -> Sum1/2, Kp_c/1
  Kp_c/1 -> Add/3
  Sum2/1 -> Ka_c/1
  Ki_c/1 -> Integrator/1
  Add/1 -> Sum2/2, Saturation/1

== system hw3/Subsystem5/DC_Motor ==
  Input_voltage : Inport
  Back EMF constant1 : Gain  Gain=Ke
  Gr : Gain  Gain=Gr
  Integrator1 : Integrator
  Sum1 : Sum  Inputs=|+-
  Torque constant1 : Gain  Gain=Kt
  Transfer Fcn1 : TransferFcn  Denominator=[La Ra]
  Transfer Fcn3 : TransferFcn  Denominator=[Jeq Beq]
  Motor_Speed(rad/s) : Outport  VectorParamsAs1DForOutWhenUnconnected=off
  Load_Speed(rad/s) : Outport  Port=2  VectorParamsAs1DForOutWhenUnconnected=off
  Load_Angle(rad) : Outport  Port=3  VectorParamsAs1DForOutWhenUnconnected=off
  Current_measurement : Outport  Port=4  VectorParamsAs1DForOutWhenUnconnected=off
  wires:
  Transfer Fcn3/1 -> Back EMF constant1/1, Gr/1, Motor_Speed(rad/s)/1
  Integrator1/1 -> Load_Angle(rad)/1
  Gr/1 -> Integrator1/1, Load_Speed(rad/s)/1
  Input_voltage/1 -> Sum1/1
  Sum1/1 -> Transfer Fcn1/1
  Transfer Fcn1/1 -> Current_measurement/1, Torque constant1/1
  Back EMF constant1/1 -> Sum1/2
  Torque constant1/1 -> Transfer Fcn3/1

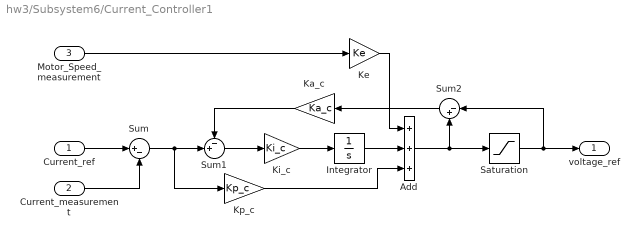
== system hw3/Subsystem6/Current_Controller1 ==
  Current_ref : Inport
  Current_measurement : Inport  Port=2
  Motor_Speed_measurement : Inport  Port=3
  Add : Sum  Inputs=+++
  Integrator : Integrator
  Ka_c : Gain  Gain=Ka_c
  Ke : Gain  Gain=Ke
  Ki_c : Gain  Gain=Ki_c
  Kp_c : Gain  Gain=Kp_c
  Saturation : Saturate  UpperLimit=48  LowerLimit=-48
  Sum : Sum  Inputs=|+-
  Sum1 : Sum  Inputs=-+|
  Sum2 : Sum  Inputs=|-+
  voltage_ref : Outport  VectorParamsAs1DForOutWhenUnconnected=off
  wires:
  Add/1 -> Saturation/1, Sum2/2
  Ki_c/1 -> Integrator/1
  Sum2/1 -> Ka_c/1
  Kp_c/1 -> Add/3
  Sum/1 -> Kp_c/1, Sum1/2
  Integrator/1 -> Add/2
  Sum1/1 -> Ki_c/1
  Current_measurement/1 -> Sum/2
  Current_ref/1 -> Sum/1
  Ka_c/1 -> Sum1/1
  Motor_Speed_measurement/1 -> Ke/1
  Ke/1 -> Add/1
  Saturation/1 -> voltage_ref/1, Sum2/1

== system hw3/Subsystem6/DC_Motor1 ==
  Input_voltage : Inport
  Back EMF constant1 : Gain  Gain=Ke
  Gr : Gain  Gain=Gr
  Integrator1 : Integrator
  Sum1 : Sum  Inputs=|+-
  Torque constant1 : Gain  Gain=Kt
  Transfer Fcn1 : TransferFcn  Denominator=[La Ra]
  Transfer Fcn3 : TransferFcn  Denominator=[Jeq Beq]
  Motor_Speed(rad/s) : Outport  VectorParamsAs1DForOutWhenUnconnected=off
  Load_Speed(rad/s) : Outport  Port=2  VectorParamsAs1DForOutWhenUnconnected=off
  Load_Angle(rad) : Outport  Port=3  VectorParamsAs1DForOutWhenUnconnected=off
  Current_measurement : Outport  Port=4  VectorParamsAs1DForOutWhenUnconnected=off
  wires:
  Torque constant1/1 -> Transfer Fcn3/1
  Back EMF constant1/1 -> Sum1/2
  Transfer Fcn1/1 -> Torque constant1/1, Current_measurement/1
  Sum1/1 -> Transfer Fcn1/1
  Input_voltage/1 -> Sum1/1
  Gr/1 -> Load_Speed(rad/s)/1, Integrator1/1
  Integrator1/1 -> Load_Angle(rad)/1
  Transfer Fcn3/1 -> Motor_Speed(rad/s)/1, Gr/1, Back EMF constant1/1

== system hw3/Subsystem6/Speed_Controller1 ==
  Load_Speed_ref : Inport
  Load_Speed_measurement : Inport  Port=2
  Add : Sum
  Integrator : Integrator
  Ka_s : Gain  Gain=Ka_s
  Ki_s : Gain  Gain=Ki_s
  Kp_s : Gain  Gain=Kp_s
  Saturation : Saturate  UpperLimit=27.3  LowerLimit=-27.3
  Sum : Sum  Inputs=|+-
  Sum1 : Sum  Inputs=-+|
  Sum2 : Sum  Inputs=|-+
  Current_ref : Outport  VectorParamsAs1DForOutWhenUnconnected=off
  wires:
  Sum/1 -> Kp_s/1, Sum1/2
  Kp_s/1 -> Add/2
  Load_Speed_ref/1 -> Sum/1
  Add/1 -> Sum2/2, Saturation/1
  Sum2/1 -> Ka_s/1
  Ka_s/1 -> Sum1/1
  Load_Speed_measurement/1 -> Sum/2
  Saturation/1 -> Current_ref/1, Sum2/1
  Ki_s/1 -> Integrator/1
  Sum1/1 -> Ki_s/1
  Integrator/1 -> Add/1

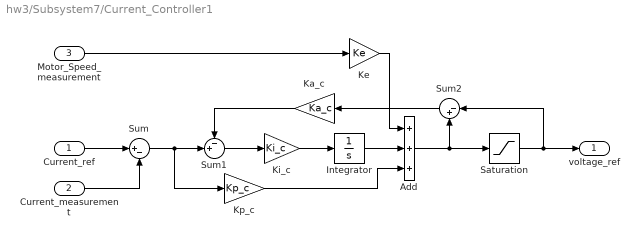
== system hw3/Subsystem7/Current_Controller1 ==
  Current_ref : Inport
  Current_measurement : Inport  Port=2
  Motor_Speed_measurement : Inport  Port=3
  Add : Sum  Inputs=+++
  Integrator : Integrator
  Ka_c : Gain  Gain=Ka_c
  Ke : Gain  Gain=Ke
  Ki_c : Gain  Gain=Ki_c
  Kp_c : Gain  Gain=Kp_c
  Saturation : Saturate  UpperLimit=48  LowerLimit=-48
  Sum : Sum  Inputs=|+-
  Sum1 : Sum  Inputs=-+|
  Sum2 : Sum  Inputs=|-+
  voltage_ref : Outport  VectorParamsAs1DForOutWhenUnconnected=off
  wires:
  Saturation/1 -> Sum2/1, voltage_ref/1
  Ke/1 -> Add/1
  Motor_Speed_measurement/1 -> Ke/1
  Ka_c/1 -> Sum1/1
  Current_ref/1 -> Sum/1
  Current_measurement/1 -> Sum/2
  Sum1/1 -> Ki_c/1
  Integrator/1 -> Add/2
  Sum/1 -> Sum1/2, Kp_c/1
  Kp_c/1 -> Add/3
  Sum2/1 -> Ka_c/1
  Ki_c/1 -> Integrator/1
  Add/1 -> Sum2/2, Saturation/1

== system hw3/Subsystem7/DC_Motor1 ==
  Input_voltage : Inport
  Back EMF constant1 : Gain  Gain=Ke
  Gr : Gain  Gain=Gr
  Integrator1 : Integrator
  Sum1 : Sum  Inputs=|+-
  Torque constant1 : Gain  Gain=Kt
  Transfer Fcn1 : TransferFcn  Denominator=[La Ra]
  Transfer Fcn3 : TransferFcn  Denominator=[Jeq Beq]
  Motor_Speed(rad/s) : Outport  VectorParamsAs1DForOutWhenUnconnected=off
  Load_Speed(rad/s) : Outport  Port=2  VectorParamsAs1DForOutWhenUnconnected=off
  Load_Angle(rad) : Outport  Port=3  VectorParamsAs1DForOutWhenUnconnected=off
  Current_measurement : Outport  Port=4  VectorParamsAs1DForOutWhenUnconnected=off
  wires:
  Transfer Fcn3/1 -> Back EMF constant1/1, Gr/1, Motor_Speed(rad/s)/1
  Integrator1/1 -> Load_Angle(rad)/1
  Gr/1 -> Integrator1/1, Load_Speed(rad/s)/1
  Input_voltage/1 -> Sum1/1
  Sum1/1 -> Transfer Fcn1/1
  Transfer Fcn1/1 -> Current_measurement/1, Torque constant1/1
  Back EMF constant1/1 -> Sum1/2
  Torque constant1/1 -> Transfer Fcn3/1

== system hw3/Subsystem7/Speed_Controller1 ==
  Load_Speed_ref : Inport
  Load_Speed_measurement : Inport  Port=2
  Add : Sum
  Integrator : Integrator
  Ka_s : Gain  Gain=Ka_s
  Ki_s : Gain  Gain=Ki_s
  Kp_s : Gain  Gain=Kp_s
  Saturation : Saturate  UpperLimit=27.3  LowerLimit=-27.3
  Sum : Sum  Inputs=|+-
  Sum1 : Sum  Inputs=-+|
  Sum2 : Sum  Inputs=|-+
  Current_ref : Outport  VectorParamsAs1DForOutWhenUnconnected=off
  wires:
  Integrator/1 -> Add/1
  Sum1/1 -> Ki_s/1
  Ki_s/1 -> Integrator/1
  Saturation/1 -> Sum2/1, Current_ref/1
  Load_Speed_measurement/1 -> Sum/2
  Ka_s/1 -> Sum1/1
  Sum2/1 -> Ka_s/1
  Add/1 -> Saturation/1, Sum2/2
  Load_Speed_ref/1 -> Sum/1
  Kp_s/1 -> Add/2
  Sum/1 -> Sum1/2, Kp_s/1

== system hw3/Subsystem8/Current_Controller1 ==
  Current_ref : Inport
  Current_measurement : Inport  Port=2
  Motor_Speed_measurement : Inport  Port=3
  Add : Sum  Inputs=+++
  Integrator : Integrator
  Ka_c : Gain  Gain=Ka_c
  Ke : Gain  Gain=Ke
  Ki_c : Gain  Gain=Ki_c
  Kp_c : Gain  Gain=Kp_c
  Saturation : Saturate  UpperLimit=48  LowerLimit=-48
  Sum : Sum  Inputs=|+-
  Sum1 : Sum  Inputs=-+|
  Sum2 : Sum  Inputs=|-+
  voltage_ref : Outport  VectorParamsAs1DForOutWhenUnconnected=off
  wires:
  Add/1 -> Saturation/1, Sum2/2
  Ki_c/1 -> Integrator/1
  Sum2/1 -> Ka_c/1
  Kp_c/1 -> Add/3
  Sum/1 -> Kp_c/1, Sum1/2
  Integrator/1 -> Add/2
  Sum1/1 -> Ki_c/1
  Current_measurement/1 -> Sum/2
  Current_ref/1 -> Sum/1
  Ka_c/1 -> Sum1/1
  Motor_Speed_measurement/1 -> Ke/1
  Ke/1 -> Add/1
  Saturation/1 -> voltage_ref/1, Sum2/1

== system hw3/Subsystem8/DC_Motor1 ==
  Input_voltage : Inport
  Back EMF constant1 : Gain  Gain=Ke
  Gr : Gain  Gain=Gr
  Integrator1 : Integrator
  Sum1 : Sum  Inputs=|+-
  Torque constant1 : Gain  Gain=Kt
  Transfer Fcn1 : TransferFcn  Denominator=[La Ra]
  Transfer Fcn3 : TransferFcn  Denominator=[Jeq Beq]
  Motor_Speed(rad/s) : Outport  VectorParamsAs1DForOutWhenUnconnected=off
  Load_Speed(rad/s) : Outport  Port=2  VectorParamsAs1DForOutWhenUnconnected=off
  Load_Angle(rad) : Outport  Port=3  VectorParamsAs1DForOutWhenUnconnected=off
  Current_measurement : Outport  Port=4  VectorParamsAs1DForOutWhenUnconnected=off
  wires:
  Torque constant1/1 -> Transfer Fcn3/1
  Back EMF constant1/1 -> Sum1/2
  Transfer Fcn1/1 -> Torque constant1/1, Current_measurement/1
  Sum1/1 -> Transfer Fcn1/1
  Input_voltage/1 -> Sum1/1
  Gr/1 -> Load_Speed(rad/s)/1, Integrator1/1
  Integrator1/1 -> Load_Angle(rad)/1
  Transfer Fcn3/1 -> Motor_Speed(rad/s)/1, Gr/1, Back EMF constant1/1

== system hw3/Subsystem8/Speed_Controller1 ==
  Load_Speed_ref : Inport
  Load_Speed_measurement : Inport  Port=2
  Add : Sum
  Integrator : Integrator
  Ka_s : Gain  Gain=Ka_s
  Ki_s : Gain  Gain=Ki_s
  Kp_s : Gain  Gain=Kp_s
  Saturation : Saturate  UpperLimit=27.3  LowerLimit=-27.3
  Sum : Sum  Inputs=|+-
  Sum1 : Sum  Inputs=-+|
  Sum2 : Sum  Inputs=|-+
  Current_ref : Outport  VectorParamsAs1DForOutWhenUnconnected=off
  wires:
  Sum/1 -> Kp_s/1, Sum1/2
  Kp_s/1 -> Add/2
  Load_Speed_ref/1 -> Sum/1
  Add/1 -> Sum2/2, Saturation/1
  Sum2/1 -> Ka_s/1
  Ka_s/1 -> Sum1/1
  Load_Speed_measurement/1 -> Sum/2
  Saturation/1 -> Current_ref/1, Sum2/1
  Ki_s/1 -> Integrator/1
  Sum1/1 -> Ki_s/1
  Integrator/1 -> Add/1

== system hw3/Subsystem9/Current_Controller2 ==
  Current_ref : Inport
  Current_measurement : Inport  Port=2
  Motor_Speed_measurement : Inport  Port=3
  Add : Sum  Inputs=+++
  Integrator : Integrator
  Ka_c : Gain  Gain=Ka_c
  Ke : Gain  Gain=Ke
  Ki_c : Gain  Gain=Ki_c
  Kp_c : Gain  Gain=Kp_c
  Saturation : Saturate  UpperLimit=48  LowerLimit=-48
  Sum : Sum  Inputs=|+-
  Sum1 : Sum  Inputs=-+|
  Sum2 : Sum  Inputs=|-+
  voltage_ref : Outport  VectorParamsAs1DForOutWhenUnconnected=off
  wires:
  Saturation/1 -> Sum2/1, voltage_ref/1
  Ke/1 -> Add/1
  Motor_Speed_measurement/1 -> Ke/1
  Ka_c/1 -> Sum1/1
  Current_ref/1 -> Sum/1
  Current_measurement/1 -> Sum/2
  Sum1/1 -> Ki_c/1
  Integrator/1 -> Add/2
  Sum/1 -> Sum1/2, Kp_c/1
  Kp_c/1 -> Add/3
  Sum2/1 -> Ka_c/1
  Ki_c/1 -> Integrator/1
  Add/1 -> Sum2/2, Saturation/1

== system hw3/Subsystem9/DC_Motor2 ==
  Input_voltage : Inport
  Back EMF constant1 : Gain  Gain=Ke
  Gr : Gain  Gain=Gr
  Integrator1 : Integrator
  Sum1 : Sum  Inputs=|+-
  Torque constant1 : Gain  Gain=Kt
  Transfer Fcn1 : TransferFcn  Denominator=[La Ra]
  Transfer Fcn3 : TransferFcn  Denominator=[Jeq Beq]
  Motor_Speed(rad/s) : Outport  VectorParamsAs1DForOutWhenUnconnected=off
  Load_Speed(rad/s) : Outport  Port=2  VectorParamsAs1DForOutWhenUnconnected=off
  Load_Angle(rad) : Outport  Port=3  VectorParamsAs1DForOutWhenUnconnected=off
  Current_measurement : Outport  Port=4  VectorParamsAs1DForOutWhenUnconnected=off
  wires:
  Transfer Fcn3/1 -> Back EMF constant1/1, Gr/1, Motor_Speed(rad/s)/1
  Integrator1/1 -> Load_Angle(rad)/1
  Gr/1 -> Integrator1/1, Load_Speed(rad/s)/1
  Input_voltage/1 -> Sum1/1
  Sum1/1 -> Transfer Fcn1/1
  Transfer Fcn1/1 -> Current_measurement/1, Torque constant1/1
  Back EMF constant1/1 -> Sum1/2
  Torque constant1/1 -> Transfer Fcn3/1

== system hw3/Subsystem9/Position_Controller2 ==
  Load_Angle_ref : Inport
  Load_Angle_measurement : Inport  Port=2
  Add : Sum
  Derivative : Derivative
  Kd_p : Gain  Gain=Kd_p
  Kp_p : Gain  Gain=Kp_p
  Saturation : Saturate  UpperLimit=6140*pi/30  LowerLimit=-6140*pi/30
  Sum : Sum  Inputs=|+-
  Load_Speed_ref : Outport  VectorParamsAs1DForOutWhenUnconnected=off
  wires:
  Add/1 -> Saturation/1
  Derivative/1 -> Add/2
  Sum/1 -> Kd_p/1, Kp_p/1
  Saturation/1 -> Load_Speed_ref/1
  Kp_p/1 -> Add/1
  Kd_p/1 -> Derivative/1
  Load_Angle_ref/1 -> Sum/1
  Load_Angle_measurement/1 -> Sum/2
